simulink model "Inverted_Pendulum"  (R2019b)
settings: Solver=ode4  StartTime=0.0  StopTime=25  FixedStep=Ts  RelTol=1e-3
values from neighbouring files (symbols this model uses):
  KK = [KK 0]    [Initialisation.m]
  sys_ss2 = c2d(sysac,T_sample)    [Initialisation.m]
  T_dist = -75    [Initialisation.m]
  T_sample = 0.01    [Initialisation.m]
  T_sat = 20    [Initialisation.m]
  x_init = [Angle_start_up; Angular_velocity_start_up]    [Initialisation.m]
undefined symbols (not defined in the file or in its folder): Discrete, Plant1, Time
libraries: simulink x2, ctrlSharedLib x1, eeLuenbergerObserver x1
settings Model: Creator=LENOVO  LastModifiedBy=dipsb
settings SolverCC: AlgebraicLoopSolver=LineSearch

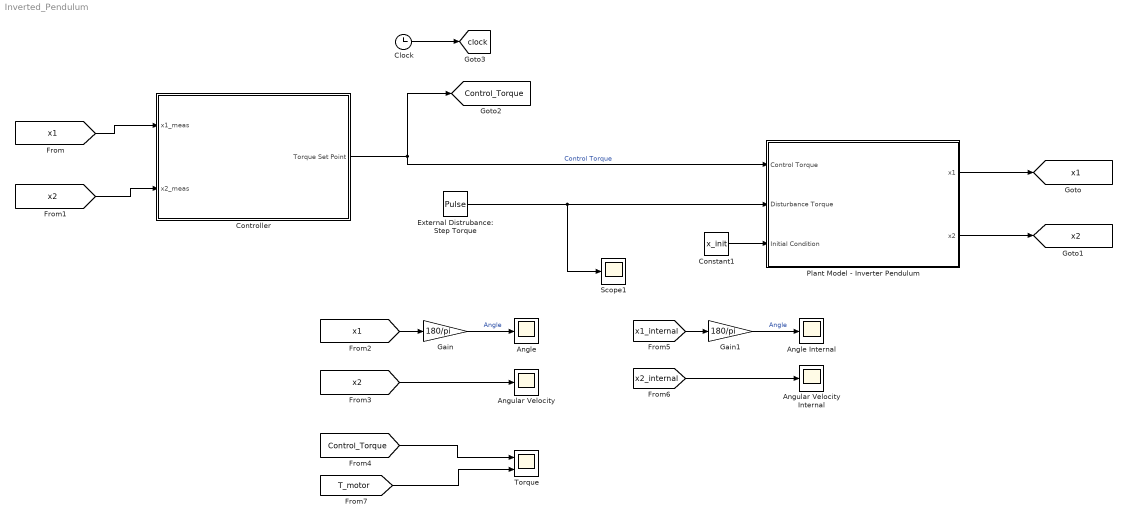
== system Inverted_Pendulum ==
  Angle : Scope
  Angle Internal : Scope
  Angular Velocity : Scope
  Angular Velocity Internal : Scope
  Clock : Clock
  Constant1 : Constant  Value=x_init
  Controller : Subsystem
  External Distrubance: Step Torque : DiscretePulseGenerator  PulseType=Time based  Amplitude=T_dist  Period=10  PulseWidth=0.1  PhaseDelay=6
  Gain : Gain  Gain=180/pi
  Gain1 : Gain  Gain=180/pi
  Plant Model - Inverter Pendulum : Subsystem  mask{Plant=Plant1}
      mask prompts: Plant "Plant structure"
      mask DialogControl DescTextVar Prompt: Contains the plant model of compound pendulum. The input below accepts the plant parameters as a structure.
  Scope1 : Scope
  Torque : Scope  NumInputPorts=2
  tag scope: Control_Torque=global, clock=global, x1=global, x2=global
  wires:
  Plant Model - Inverter Pendulum/1(x1) -> [x1]
  Plant Model - Inverter Pendulum/2(x2) -> [x2]
  [x1] -> Controller/1(x1_meas)
  [x2] -> Controller/2(x2_meas)
  Controller/1("Torque Set Point ") -> Plant Model - Inverter Pendulum/1(Control Torque), [Control_Torque]  "Control Torque"
  [x1] -> Gain/1
  Gain/1 -> Angle/1  "Angle"
  [x2] -> Angular Velocity/1
  Clock/1 -> [clock]
  Constant1/1 -> Plant Model - Inverter Pendulum/3(Initial Condition)
  Gain1/1 -> Angle Internal/1  "Angle"
  [x1_internal] -> Gain1/1
  [x2_internal] -> Angular Velocity Internal/1
  [T_motor] -> Torque/2
  [Control_Torque] -> Torque/1
  External Distrubance: Step Torque/1 -> Plant Model - Inverter Pendulum/2(Disturbance Torque), Scope1/1

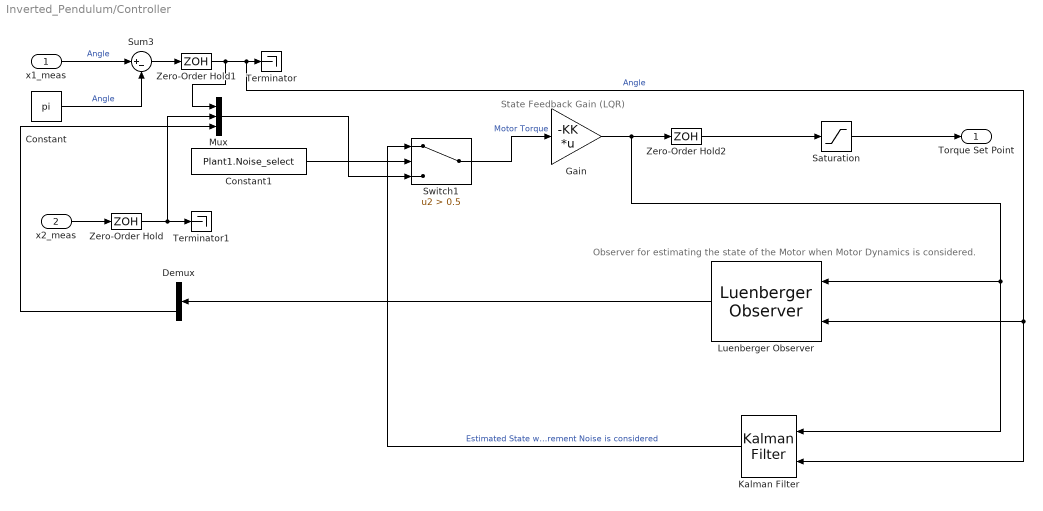
== system Inverted_Pendulum/Controller ==
  note: State Feedback Gain (LQR)
  note: Observer for estimating the state of the Motor when Motor Dynamics is considered.
  x1_meas : Inport
  x2_meas : Inport  Port=2
  Constant : Constant  Value=pi
  Constant1 : Constant  Value=Plant1.Noise_select
  Demux : Demux  Outputs=3
  Gain : Gain  Gain=-KK  Multiplication=Matrix(K*u)
  Kalman Filter : ctrlSharedLib/Kalman Filter  TimeDomain=Discrete-Time  UseCurrentEstimator=on  ModelSource=Individual A, B, C, D matrices  ModelSourceVariable=ss(0.95,1,1,0,1)  A=sys_ss2.A  B=sys_ss2.B  C=sys_ss2.C  D=sys_ss2.D  NumberOfStates=1  NumberOfInputs=1  NumberOfOutputs=1  InitialEstimateSource=Dialog  X0=[0 0 0]  P0=10  UseK=off  UseGH=off  NumberOfProcessNoiseInputs=1  G=eye(3)  TimeInvariantG=on  H=0  TimeInvariantH=on  Q=0  TimeInvariantQ=on  R=1  TimeInvariantR=on  N=0  TimeInvariantN=on  AddInputPort=on  AddEnablePort=off  OutputEstimatedY=off  OutputP=off  Ts=T_sample
  Luenberger Observer : eeLuenbergerObserver/Luenberger Observer  StateSpaceType=Discrete-time  Ad=sys_ss2.A  Bd=sys_ss2.B  Cd=sys_ss2.C  Dd=sys_ss2.D  A=1  B=1  C=1  D=1  ObserverDesign=Desired eigenvalues  Ld=1  DesiredEigenvalues=[0.4 0.3 0.2]  x0=[0 0 0]  Tsd=0.1  Ts=T_sample
      settings: SourceProductBaseCode=PS
  Mux : Mux  Inputs=3
  Saturation : Saturate  UpperLimit=T_sat  LowerLimit=-T_sat
  Sum3 : Sum  Inputs=|+-
  Switch1 : Switch  Criteria=u2 > Threshold  Threshold=0.5
  Terminator : Terminator
  Terminator1 : Terminator
  Zero-Order Hold : ZeroOrderHold  SampleTime=T_sample
  Zero-Order Hold1 : ZeroOrderHold  SampleTime=T_sample
  Zero-Order Hold2 : ZeroOrderHold  SampleTime=T_sample
  "Torque Set Point " : Outport
  wires:
  x2_meas/1 -> Zero-Order Hold/1
  Zero-Order Hold/1 -> Mux/2, Terminator1/1
  x1_meas/1 -> Sum3/1  "Angle"
  Constant/1 -> Sum3/2  "Angle"
  Gain/1 -> Kalman Filter/1, Luenberger Observer/1, Zero-Order Hold2/1
  Zero-Order Hold2/1 -> Saturation/1
  Saturation/1 -> "Torque Set Point "/1
  Sum3/1 -> Zero-Order Hold1/1
  Zero-Order Hold1/1 -> Mux/1, Kalman Filter/2, Luenberger Observer/2, Terminator/1  "Angle"
  Kalman Filter/1 -> Switch1/1  "Estimated State when Measurement Noise is considered"
  Luenberger Observer/1 -> Demux/1
  Constant1/1 -> Switch1/2
  Mux/1 -> Switch1/3
  Switch1/1 -> Gain/1  "Motor Torque"
  Demux/3 -> Mux/3

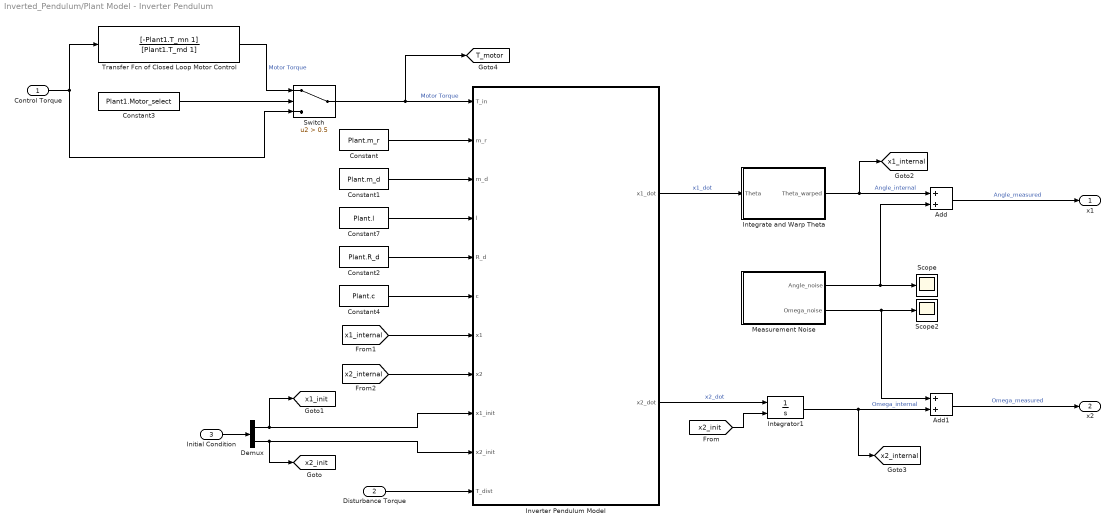
== system Inverted_Pendulum/Plant Model - Inverter Pendulum ==
  Control Torque : Inport
  Disturbance Torque : Inport  Port=2
  Initial Condition : Inport  Port=3
  Add : Sum
  Add1 : Sum
  Constant : Constant  Value=Plant.m_r
  Constant1 : Constant  Value=Plant.m_d
  Constant2 : Constant  Value=Plant.R_d
  Constant3 : Constant  Value=Plant1.Motor_select
  Constant4 : Constant  Value=Plant.c
  Constant7 : Constant  Value=Plant.l
  Demux : Demux  Outputs=2
  Integrate and Warp Theta : Subsystem
  Integrator1 : Integrator  InitialConditionSource=external
  Inverter Pendulum Model : MATLAB Function  TreatAsAtomicUnit=on
  "Measurement Noise " : Subsystem
  Scope : Scope
  Scope2 : Scope
  Switch : Switch  Criteria=u2 > Threshold  Threshold=0.5
  "Transfer Fcn of Closed Loop Motor Control " : TransferFcn  Numerator=[-Plant1.T_mn 1]  Denominator=[Plant1.T_md 1]
  x1 : Outport
  x2 : Outport  Port=2
  tag scope: T_motor=global, x1_init=global, x1_internal=global, x2_init=global, x2_internal=global
  wires:
  Inverter Pendulum Model/2(x2_dot) -> Integrator1/1  "x2_dot"
  Control Torque/1 -> Switch/3, "Transfer Fcn of Closed Loop Motor Control "/1
  Integrator1/1 -> [x2_internal], Add1/2  "Omega_internal"
  Constant/1 -> Inverter Pendulum Model/2(m_r)
  Constant1/1 -> Inverter Pendulum Model/3(m_d)
  Constant7/1 -> Inverter Pendulum Model/4(l)
  Demux/2 -> Inverter Pendulum Model/10(x2_init), [x2_init]
  Constant4/1 -> Inverter Pendulum Model/6(c)
  Constant2/1 -> Inverter Pendulum Model/5(R_d)
  [x2_init] -> Integrator1/2
  Integrate and Warp Theta/1(Theta_warped) -> [x1_internal], Add/1  "Angle_internal"
  Inverter Pendulum Model/1(x1_dot) -> Integrate and Warp Theta/1(Theta)  "x1_dot"
  Disturbance Torque/1 -> Inverter Pendulum Model/11(T_dist)
  Initial Condition/1 -> Demux/1
  Demux/1 -> Inverter Pendulum Model/9(x1_init), [x1_init]
  Add/1 -> x1/1  "Angle_measured"
  Add1/1 -> x2/1  "Omega_measured"
  [x1_internal] -> Inverter Pendulum Model/7(x1)
  [x2_internal] -> Inverter Pendulum Model/8(x2)
  "Measurement Noise "/1(Angle_noise) -> Add/2, Scope/1
  "Measurement Noise "/2(Omega_noise) -> Add1/1, Scope2/1
  Switch/1 -> [T_motor], Inverter Pendulum Model/1(T_in)  "Motor Torque"
  "Transfer Fcn of Closed Loop Motor Control "/1 -> Switch/1  "Motor Torque"
  Constant3/1 -> Switch/2

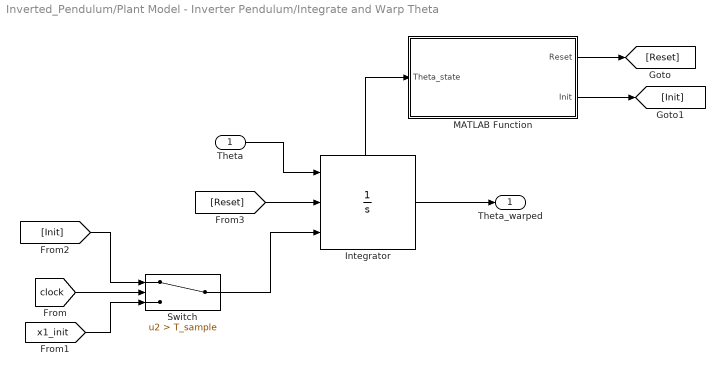
== system Inverted_Pendulum/Plant Model - Inverter Pendulum/Integrate and Warp Theta ==
  Theta : Inport
  Integrator : Integrator  ExternalReset=rising  InitialConditionSource=external  ShowStatePort=on
  MATLAB Function : MATLAB Function  TreatAsAtomicUnit=on
  Switch : Switch  Criteria=u2 > Threshold  Threshold=T_sample
  Theta_warped : Outport
  wires:
  Theta/1 -> Integrator/1
  Integrator/1 -> Theta_warped/1
  [x1_init] -> Switch/3
  [clock] -> Switch/2
  Switch/1 -> Integrator/3
  Integrator/State -> MATLAB Function/1(Theta_state)
  MATLAB Function/1(Reset) -> [Reset]
  MATLAB Function/2(Init) -> [Init]
  [Init] -> Switch/1
  [Reset] -> Integrator/2

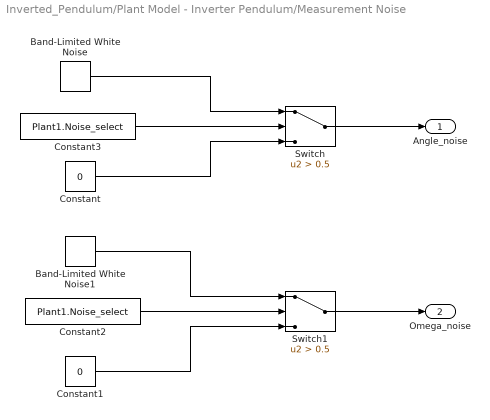
== system Inverted_Pendulum/Plant Model - Inverter Pendulum/Measurement Noise  ==
  Band-Limited White Noise : simulink/Sources/Band-Limited White Noise  Cov=1e-6  Ts=T_sample  seed=[23341]
  Band-Limited White Noise1 : simulink/Sources/Band-Limited White Noise  Cov=1e-5  Ts=T_sample  seed=[23341]
  Constant : Constant  Value=0
  Constant1 : Constant  Value=0
  Constant2 : Constant  Value=Plant1.Noise_select
  Constant3 : Constant  Value=Plant1.Noise_select
  Switch : Switch  Criteria=u2 > Threshold  Threshold=0.5
  Switch1 : Switch  Criteria=u2 > Threshold  Threshold=0.5
  Angle_noise : Outport
  Omega_noise : Outport  Port=2
  wires:
  Constant3/1 -> Switch/2
  Switch/1 -> Angle_noise/1
  Band-Limited White Noise/1 -> Switch/1
  Constant/1 -> Switch/3
  Switch1/1 -> Omega_noise/1
  Band-Limited White Noise1/1 -> Switch1/1
  Constant1/1 -> Switch1/3
  Constant2/1 -> Switch1/2

== matlab function Inverted_Pendulum/Plant Model - Inverter Pendulum/Integrate and Warp Theta/MATLAB Function ==
  data: Theta_state input; Reset output; Init output
function [Reset, Init] = fcn(Theta_state)
Reset = 0;
Init = 0;
if Theta_state >= 2*pi
    Init = 2*pi - Theta_state;
    Reset = 1;
end
if Theta_state < 0 
    Init = 2*pi + Theta_state;
    Reset = 1;
end

== matlab function Inverted_Pendulum/Plant Model - Inverter Pendulum/Inverter Pendulum Model ==
  settings: updateMethod=DISCRETE
  data: T_in input; x1_dot output; m_r input; m_d input; l input; R_d input; c input; x1 input; x2 input; x1_init input; x2_init input; x2_dot output; T_dist input
function [x1_dot,x2_dot] = Inverted_Pendulum(T_in, m_r, m_d, l, R_d, c, x1, x2, x1_init, x2_init, T_dist)

% T_in  - Input variable - control torque [Nm]
% m_r   - Mass of the rod [Kg]
% m_d   - Mass of the disc [Kg]
% l     - Length of the rod [m]
% R_d   - Radius of circular disc [m]
% c     - Coefficient of air friction []
% T_dist- Disturbance Torque [Nm]

% x1    - State Variable -  Angle of deviation [rad], 0 radians correspond to downward
% position

% x2    - State Variable - Angular velocity [rad/s]

% x1_dot - Derivative of state x1 - Angular velocity [rad/s]

% x2_dot - Derivative of state x1 - Angular acceleration [rad/s^2]

g = 9.81;  % acceleration due to gravity [m/s^2]
J = (m_r/3 + m_d)*l^2 + m_d*R_d^2/2 ; % Inertia of the compund pendulum [Kg m^2]


persistent flag;

if isempty(flag)   % Setting initial conditions to x1 and x2 at the start of simulation
    x1 = x1_init;
    x2 = x2_init;
    flag = 1;
end


x1_dot = x2;                                              % First State Equation

x2_dot = -(m_r/2 + m_d)*g*l*sin(x1)/J - c*x2/J + T_in/J + T_dist/J;  % Second State Equation 

end
